simulink model "PIDRoiRac"  (R2014a)
settings: Solver=ode8  StartTime=0.0  StopTime=10  FixedStep=T  RelTol=1e-3
undefined symbols (not defined in the file or in its folder): Kp, T
settings Model: Creator=tri  LastModifiedBy=tri

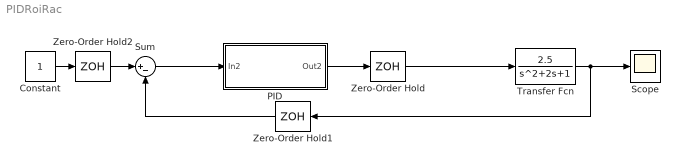
== system PIDRoiRac ==
  Constant : Constant
  PID : Subsystem
  Scope : Scope
  Sum : Sum  Inputs=|+-
  Transfer Fcn : TransferFcn  Numerator=[2.5]
  Zero-Order Hold : ZeroOrderHold
  Zero-Order Hold1 : ZeroOrderHold
  Zero-Order Hold2 : ZeroOrderHold
  wires:
  Sum/1 -> PID/1(In2)
  Constant/1 -> Zero-Order Hold2/1
  PID/1(Out2) -> Zero-Order Hold/1
  Transfer Fcn/1 -> Zero-Order Hold1/1, Scope/1
  Zero-Order Hold/1 -> Transfer Fcn/1
  Zero-Order Hold1/1 -> Sum/2
  Zero-Order Hold2/1 -> Sum/1

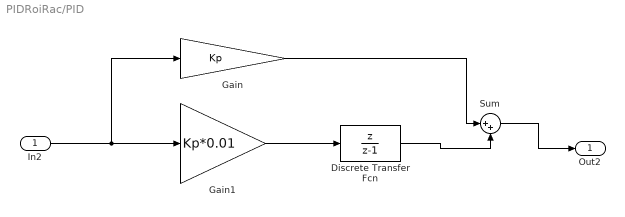
== system PIDRoiRac/PID ==
  In2 : Inport
  Discrete Transfer Fcn : DiscreteTransferFcn  Numerator=[1 0 ]  Denominator=[1 -1]  SampleTime=T
  Gain : Gain  Gain=Kp
  Gain1 : Gain  Gain=Kp*0.01
  Sum : Sum  Inputs=|++
  Out2 : Outport
  wires:
  Gain1/1 -> Discrete Transfer Fcn/1
  In2/1 -> Gain/1, Gain1/1
  Discrete Transfer Fcn/1 -> Sum/2
  Gain/1 -> Sum/1
  Sum/1 -> Out2/1
